simulink model "PI_v3"  (R2022b)
settings: Solver=FixedStepAuto  StartTime=0.0  StopTime=250  FixedStep=0.1  RelTol=1e-3  EnableMultiTasking=on
InitFcn:
  | Ts = 0.1
values from neighbouring files (symbols this model uses):
  ki = 10^controllerParams(2)    [objFunDreitankt.m]
  kp = 10^controllerParams(1)    [objFunDreitankt.m]
  tstart = min(simout.enableControl.time(simout.enableControl.signals.values > 0.5))    [objFunDreitankt.m]
  upperBound1stank = 7.5*10^-3    (= 0.0075)    [objFunDreitankt.m]
  V101_ref = 0    [objFunDreitankt.m]
undefined symbols (not defined in the file or in its folder): ESSettings, f, Parameters
libraries: etargetslib x134, simulink x32, instrumentlib x2, pid_lib x1, slpidlib x1, UtilLib x1
settings Model: Creator=ST  LastModifiedBy=vd818225
settings SolverCC: ZeroCrossAlgorithm=Adaptive  AlgebraicLoopSolver=TrustRegion  AutoInsertRateTranBlk=on
settings DataIOCC: LimitDataPoints=on  SaveFormat=Array  ReturnWorkspaceOutputs=off
settings OptimizationCC: LifeSpan=inf
settings DebuggingCC: UnderspecifiedInitializationDetection=Classic  MergeDetectMultiDrivingBlocksExec=none  SolverPrmCheckMsg=warning  UnconnectedInputMsg=warning  UnconnectedOutputMsg=warning  UnconnectedLineMsg=warning  StateNameClashWarn=warning  SFUnexpectedBacktrackingDiag=warning  SFNoUnconditionalDefaultTransitionDiag=warning  SFExecutionAtInitializationDiag=none  SFMachineParentedDataDiag=warning  ArithmeticOperatorsInVariantConditions=warning
settings HardwareCC: ProdBitPerPointer=32  ProdBitPerSizeT=32  ProdBitPerPtrDiffT=32  ProdLargestAtomicFloat=None  ProdIntDivRoundTo=Undefined  ProdEndianess=Unspecified  ProdWordSize=32  ProdHWDeviceType=32-bit Generic
settings ModelReferenceCC: EnableRefExpFcnMdlSchedulingChecks=on  PropagateSignalLabelsOutOfModel=off
settings SFSimCC: SimUseLocalCustomCode=off  CustomCodeUndefinedFunction=UseInterfaceOnly
settings RTWCC: RTWUseLocalCustomCode=off  DLArmComputeVersion=19.05
settings CodeAppCC: StateflowObjectComments=on
settings GRTTargetCC: TargetLangStandard=C89/C90 (ANSI)
settings ConfigComp: CovMetricSettings=dw  CovSaveCumulativeToWorkspaceVar=on  CovSaveSingleToWorkspaceVar=on  CovExternalEMLEnable=off  CovSFcnEnable=off

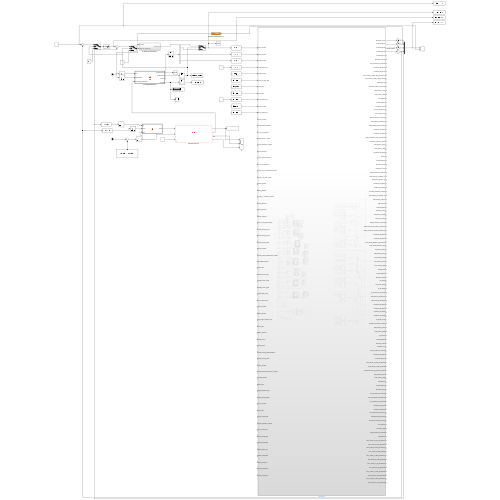
[thumbnail: Simulink's stored preview of the top-level diagram]
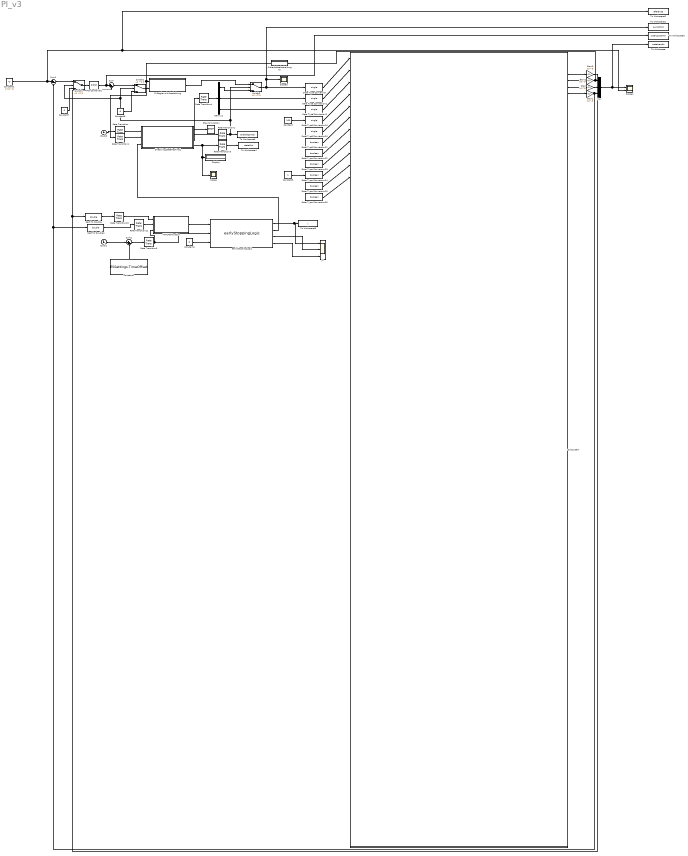
== system PI_v3 ==
  Cast To Double : DataTypeConversion  OutDataTypeStr=double  SaturateOnIntegerOverflow=off  RndMeth=Floor
  Cast To Double1 : DataTypeConversion  OutDataTypeStr=double  SaturateOnIntegerOverflow=off  RndMeth=Floor
  Clock1 : Clock
  Clock3 : Clock
  Constant : Constant  Value=100
  Constant1 : Constant  Value=4*10^-3
  Constant2 : Constant  Value=ESSettings.TimeOffset
  Constant3 : Constant
  Constant4 : Constant  Value=0
  Constant7 : Constant  Value=0
  Constant8 : Constant  Value=0
  Data Type Conversion{,1..2,19..20} (5 alike) : DataTypeConversion  OutDataTypeStr=single  SaturateOnIntegerOverflow=off  RndMeth=Floor
  Data Type Conversion{21..26} (6 alike) : DataTypeConversion  OutDataTypeStr=boolean  SaturateOnIntegerOverflow=off  RndMeth=Floor
  Demux1 : Demux  Outputs=3
  Display : Display
  Gain : Gain  Gain=10^-3
  Gain1 : Gain  Gain=10^-3
  Gain2 : Gain  Gain=10^-3
  Gain3 : Gain  Gain=10^-5
  J1 : Scope  NumInputPorts=3
  MATLAB Function : MATLAB Function  TreatAsAtomicUnit=on
  Mux : Mux  Inputs=3
  PI-Regler mit Abschaltung : Subsystem
  PID Controller1 : slpidlib/PID Controller  Controller=PID  Form=Parallel  TimeDomain=Continuous-time  UseExternalTs=off  SampleTime=-1  IntegratorMethod=Forward Euler  FilterMethod=Forward Euler  ControllerParametersSource=internal  P=kp  I=ki  UseKiTs=off  D=0  N=100  UseFilter=on  TunerSelectOption=Transfer Function Based (PID Tuner App)  InitialConditionSource=internal  InitialConditionForIntegrator=0  InitialConditionForFilter=0  DifferentiatorICPrevScaledInput=0  ExternalReset=none  TrackingMode=off  Kt=1  LimitOutput=on  SatLimitsSource=internal  UpperSaturationLimit=50/60  LowerSaturationLimit=0  LinearizeAsGain=on  AntiWindupMode=clamping  Kb=1  LimitIntegrator=off  UpperIntegratorSaturationLimit=inf  LowerIntegratorSaturationLimit=-inf  POutMin=[]  POutMax=[]  IOutMin=[]  IOutMax=[]  DOutMin=[]  DOutMax=[]  NOutMin=[]  NOutMax=[]  SumOutMin=[]  SumOutMax=[]  SaturationOutMin=[]  SaturationOutMax=[]  PParamMin=[]  PParamMax=[]  IParamMin=[]  IParamMax=[]  DParamMin=[]  DParamMax=[]  NParamMin=[]  NParamMax=[]  KbParamMin=[]  KbParamMax=[]  KtParamMin=[]  KtParamMax=[]  KbOutMin=[]  KbOutMax=[]  KtOutMin=[]  KtOutMax=[]  IntegratorOutMin=[]  IntegratorOutMax=[]  FilterOutMin=[]  FilterOutMax=[]  SumI1OutMin=[]  SumI1OutMax=[]  SumI2OutMin=[]  SumI2OutMax=[]  SumI3OutMin=[]  SumI3OutMax=[]  SumI4OutMin=[]  SumI4OutMax=[]  SumDOutMin=[]  SumDOutMax=[]  DifferentiatorOutMin=[]  DifferentiatorOutMax=[]  FilterDiffOutCoefMin=[]  FilterDiffOutCoefMax=[]  ReciprocalOutMin=[]  ReciprocalOutMax=[]  SumDenOutMin=[]  SumDenOutMax=[]  SumNumOutMin=[]  SumNumOutMax=[]  DivideOutMin=[]  DivideOutMax=[]  UdiffTsProdOutMin=[]  UdiffTsProdOutMax=[]  NTsProdOutMin=[]  NTsProdOutMax=[]  UintegralTsProdOutMin=[]  UintegralTsProdOutMax=[]  UngainTsProdOutMin=[]  UngainTsProdOutMax=[]  ClampingZeroOutDataTypeStr=Inherit: Inherit via back propagation  ClampingZeroOutMin=[]  ClampingZeroOutMax=[]  FilterDenConstantOutDataTypeStr=Inherit: Inherit via back propagation  FilterDenConstantOutMin=[]  FilterDenConstantOutMax=[]  PCopyOutDataTypeStr=Inherit: Inherit via back propagation  PCopyOutMin=[]  PCopyOutMax=[]  NCopyOutDataTypeStr=Inherit: Inherit via back propagation  NCopyOutMin=[]  NCopyOutMax=[]  IntegratorContinuousStateAttributes=''  IntegratorStateMustResolveToSignalObject=off  IntegratorRTWStateStorageClass=Auto  FilterContinuousStateAttributes=''  FilterStateMustResolveToSignalObject=off  FilterRTWStateStorageClass=Auto  ParallelPVariant=InternalParameters  IdealPVariant=Disabled  IVariant=InternalParameters  DVariant=InternalParameters  IntegratorVariant=Continuous  SatVariant=Enabled  AWVariant=ContClampingParallel  PCopyVariant=Disabled  TRVariant=Disabled  FdbkBlocksVariant=Forward  IdealPFdbkVariant=Disabled  SatFdbkVariant=Disabled  DerivativeFilterVariant=ContFilter  NVariant=InternalParameters  NCopyVariant=Disabled  FilterICVariant=InternalICsFilter  IntegratorICVariant=InternalICs  ExternalResetVariant=Disabled  TRSumVariant=Passthrough  SumFdbkVariant=Disabled  SumVariant=Sum_PID  TsampFilterVariant=InternalTs  TsampNgainVariant=Passthrough  TsampIntegralVariant=Passthrough  ExternalSaturationOutDataTypeStr=Inherit: Same as second input
  Rate Transition : RateTransition  OutPortSampleTime=0.1
  Rate Transition1 : RateTransition  OutPortSampleTime=0.1
  Rate Transition10 : RateTransition  OutPortSampleTime=ESSettings.t_obj
  Rate Transition11 : RateTransition  OutPortSampleTime=ESSettings.t_obj
  Rate Transition2 : RateTransition
  Rate Transition3 : RateTransition
  Rate Transition4 : RateTransition
  Rate Transition9 : RateTransition  OutPortSampleTime=ESSettings.t_obj
  Scope : Scope
  Scope1 : Scope  NumInputPorts=2
  Scope3 : Scope
  ShedulingStateMachine1 : MATLAB Function  TreatAsAtomicUnit=on
  Sicherheitsabschaltung V2 : Subsystem
  Stop Simulation : Stop
  Subsystem : Subsystem
  Sum : Sum  Inputs=|+-
  Sum1 : Sum  Inputs=|+-
  Sum2 : Sum  Inputs=|+-
  Switch1 : Switch  Criteria=u2 ~= 0  Threshold=tstart  SaturateOnIntegerOverflow=off  InputSameDT=off
  Switch2 : Switch  Criteria=u2 ~= 0  Threshold=tstart  SaturateOnIntegerOverflow=off  InputSameDT=off
  Switch3 : Switch  Criteria=u2 ~= 0  Threshold=tstart  SaturateOnIntegerOverflow=off  InputSameDT=off
  To Workspace : ToWorkspace  VariableName=waterLevels  SaveFormat=Structure With Time  SampleTime=-1
  To Workspace1 : ToWorkspace  VariableName=pumpCmd  SaveFormat=Structure With Time  SampleTime=-1
  To Workspace2 : ToWorkspace  VariableName=reference  SaveFormat=Structure With Time  SampleTime=-1
  To Workspace3 : ToWorkspace  VariableName=outerLoopCmd  SaveFormat=Structure With Time  SampleTime=-1
  To Workspace4 : ToWorkspace  VariableName=stateOut  SaveFormat=Structure With Time  SampleTime=-1
  To Workspace5 : ToWorkspace  VariableName=enableControl  SaveFormat=Structure With Time  SampleTime=-1
  To Workspace8 : ToWorkspace  VariableName=j  SaveFormat=Structure With Time  SampleTime=-1
  earlyStoppingLogic : UtilLib/earlyStoppingLogic  SystemSampleTime=-1  VariantActivationTime=update diagram  Latency=0  AutoFrameSizeCalculation=off
  wires:
  Data Type Conversion2/1 -> Subsystem/3(V106_Stellwert)
  Data Type Conversion/1 -> Subsystem/1(P101_Stellwert)
  Data Type Conversion1/1 -> Subsystem/2(V101_Stellwert)
  Data Type Conversion19/1 -> Subsystem/4(V106_Aktivierung)
  Data Type Conversion20/1 -> Subsystem/5(P102_Stellwert)
  Data Type Conversion21/1 -> Subsystem/6(V107_zu_KMP_VBS)
  Data Type Conversion22/1 -> Subsystem/7(V101_offen)
  Data Type Conversion23/1 -> Subsystem/8(V106_offen)
  Data Type Conversion24/1 -> Subsystem/9(P101_Aktivierung)
  Data Type Conversion25/1 -> Subsystem/10(V105_zu_VBS)
  Data Type Conversion26/1 -> Subsystem/11(P102_Aktivierung)
  Sicherheitsabschaltung V2/1(Notaus) -> Rate Transition1/1, PI-Regler mit Abschaltung/1(Not-Aus)
  PID Controller1/1 -> To Workspace3/1, Sum/1
  Sum1/1 -> Switch1/1
  Constant/1 -> Data Type Conversion19/1
  Constant3/1 -> Data Type Conversion24/1
  Subsystem/4(Fuellstand_B104) -> Gain1/1
  Subsystem/3(Fuellstand_B103) -> Gain/1  "Fuellstand_B103"
  Subsystem/2(Fuellstand_B102) -> Gain2/1
  Subsystem/1(Durchfluss_FI101) -> Gain3/1
  Gain2/1 -> Sicherheitsabschaltung V2/1(V2), Mux/1
  Gain/1 -> Mux/2
  Mux/1 -> To Workspace/1, Scope1/1
  Demux1/2 -> Data Type Conversion1/1
  Switch3/1 -> Data Type Conversion/1, To Workspace1/1, Scope3/1
  Demux1/3 -> Data Type Conversion2/1
  Constant1/1 -> To Workspace2/1, Scope1/2, Sum1/1
  Constant7/1 -> Switch1/3
  Switch1/1 -> PID Controller1/1
  Switch2/1 -> PI-Regler mit Abschaltung/2(Q_P101_soll [m^3/s])
  Rate Transition2/1 -> To Workspace5/1, Switch1/2, Switch2/2, Switch3/2
  Constant8/1 -> Switch2/3
  ShedulingStateMachine1/2(enableControl) -> Rate Transition2/1
  Sum/1 -> Switch2/1
  Clock3/1 -> Rate Transition/1
  ShedulingStateMachine1/1(stopExperiment) -> Stop Simulation/1
  Demux1/1 -> Switch3/3
  ShedulingStateMachine1/4(stateOut) -> Rate Transition3/1, Scope/1, Display/1
  PI-Regler mit Abschaltung/1(U_P101 [%]) -> Switch3/1
  Rate Transition/1 -> ShedulingStateMachine1/1(time)
  Rate Transition1/1 -> ShedulingStateMachine1/2(notAusActive)
  Rate Transition3/1 -> To Workspace4/1
  ShedulingStateMachine1/3(sollVals) -> Rate Transition4/1
  Rate Transition4/1 -> Demux1/1
  Sum2/1 -> Rate Transition9/1
  Gain3/1 -> Cast To Double/1, Sum/2
  Constant4/1 -> earlyStoppingLogic/3
  Rate Transition9/1 -> MATLAB Function/3(time), earlyStoppingLogic/2
  earlyStoppingLogic/2 -> ShedulingStateMachine1/3(earlyStoppingActivated)
  earlyStoppingLogic/3 -> J1/2  "JOut"
  Rate Transition11/1 -> MATLAB Function/2(meas)
  Rate Transition10/1 -> MATLAB Function/1(ref)
  MATLAB Function/1(ITAE) -> earlyStoppingLogic/1
  Clock1/1 -> Sum2/1
  Constant2/1 -> Sum2/2
  earlyStoppingLogic/4 -> J1/3
  Gain1/1 -> Cast To Double1/1, Sum1/2, Mux/3
  earlyStoppingLogic/1 -> J1/1, To Workspace8/1
  Cast To Double/1 -> Rate Transition10/1
  Cast To Double1/1 -> Rate Transition11/1

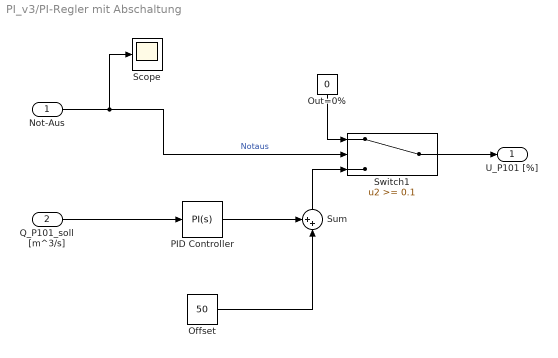
== system PI_v3/PI-Regler mit Abschaltung ==
  Not-Aus : Inport
  Q_P101_soll [m^3/s] : Inport  Port=2
  Offset : Constant  Value=50
  Out=0% : Constant  Value=0
  PID Controller : pid_lib/PID Controller  Controller=PI  Form=Parallel  TimeDomain=Continuous-time  UseExternalTs=off  SampleTime=-1  IntegratorMethod=Forward Euler  FilterMethod=Forward Euler  ControllerParametersSource=internal  P=30e3  I=0.6e3  D=0  UseFilter=on  N=100  TunerSelectOption=Transfer Function Based (PID Tuner App)  InitialConditionSource=internal  InitialConditionForIntegrator=0  InitialConditionForFilter=0  DifferentiatorICPrevScaledInput=0  ExternalReset=none  TrackingMode=off  Kt=1  LimitOutput=on  SatLimitsSource=internal  UpperSaturationLimit=50  LowerSaturationLimit=-50  LinearizeAsGain=on  AntiWindupMode=clamping  Kb=1  POutMin=[]  POutMax=[]  IOutMin=[]  IOutMax=[]  DOutMin=[]  DOutMax=[]  NOutMin=[]  NOutMax=[]  SumOutMin=[]  SumOutMax=[]  SaturationOutMin=[]  SaturationOutMax=[]  PParamMin=[]  PParamMax=[]  IParamMin=[]  IParamMax=[]  DParamMin=[]  DParamMax=[]  NParamMin=[]  NParamMax=[]  KbParamMin=[]  KbParamMax=[]  KtParamMin=[]  KtParamMax=[]  KbOutMin=[]  KbOutMax=[]  KtOutMin=[]  KtOutMax=[]  IntegratorOutMin=[]  IntegratorOutMax=[]  FilterOutMin=[]  FilterOutMax=[]  SumI1OutMin=[]  SumI1OutMax=[]  SumI2OutMin=[]  SumI2OutMax=[]  SumI3OutMin=[]  SumI3OutMax=[]  SumI4OutMin=[]  SumI4OutMax=[]  SumDOutMin=[]  SumDOutMax=[]  DifferentiatorOutMin=[]  DifferentiatorOutMax=[]  FilterDiffOutCoefMin=[]  FilterDiffOutCoefMax=[]  ReciprocalOutMin=[]  ReciprocalOutMax=[]  SumDenOutMin=[]  SumDenOutMax=[]  SumNumOutMin=[]  SumNumOutMax=[]  DivideOutMin=[]  DivideOutMax=[]  UdiffTsProdOutMin=[]  UdiffTsProdOutMax=[]  NTsProdOutMin=[]  NTsProdOutMax=[]  UintegralTsProdOutMin=[]  UintegralTsProdOutMax=[]  UngainTsProdOutMin=[]  UngainTsProdOutMax=[]  IntegratorContinuousStateAttributes=''  IntegratorStateMustResolveToSignalObject=off  IntegratorRTWStateStorageClass=Auto  FilterContinuousStateAttributes=''  FilterStateMustResolveToSignalObject=off  FilterRTWStateStorageClass=Auto  ParallelPVariant=InternalParameters  IdealPVariant=Disabled  IVariant=InternalParameters  DVariant=Disabled  IntegratorVariant=Continuous  SatVariant=Enabled  AWVariant=ContClampingParallel  PCopyVariant=Disabled  TRVariant=Disabled  FdbkBlocksVariant=Forward  IdealPFdbkVariant=Disabled  SatFdbkVariant=Disabled  DerivativeFilterVariant=Disabled  NVariant=Disabled  NCopyVariant=Disabled_SignalSpec  FilterICVariant=Disabled  IntegratorICVariant=InternalICs  ExternalResetVariant=Disabled  TRSumVariant=Passthrough  SumFdbkVariant=Disabled  SumVariant=Sum_PI  TsampFilterVariant=InternalTs  TsampNgainVariant=Passthrough  TsampIntegralVariant=Passthrough  ExternalSaturationOutDataTypeStr=Inherit: Same as second input
  Scope : Scope
  Sum : Sum  Inputs=++|
  Switch1 : Switch  Threshold=0.1
  U_P101 [%] : Outport
  wires:
  Q_P101_soll [m^3/s]/1 -> PID Controller/1
  Switch1/1 -> U_P101 [%]/1
  Out=0%/1 -> Switch1/1
  Not-Aus/1 -> Scope/1, Switch1/2  "Notaus"
  Sum/1 -> Switch1/3
  PID Controller/1 -> Sum/1
  Offset/1 -> Sum/2

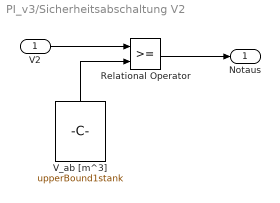
== system PI_v3/Sicherheitsabschaltung V2 ==
  V2 : Inport
  Relational Operator : RelationalOperator  InputSameDT=off
  V_ab [m^3] : Constant  Value=upperBound1stank
  Notaus : Outport
  wires:
  V2/1 -> Relational Operator/1
  V_ab [m^3]/1 -> Relational Operator/2
  Relational Operator/1 -> Notaus/1

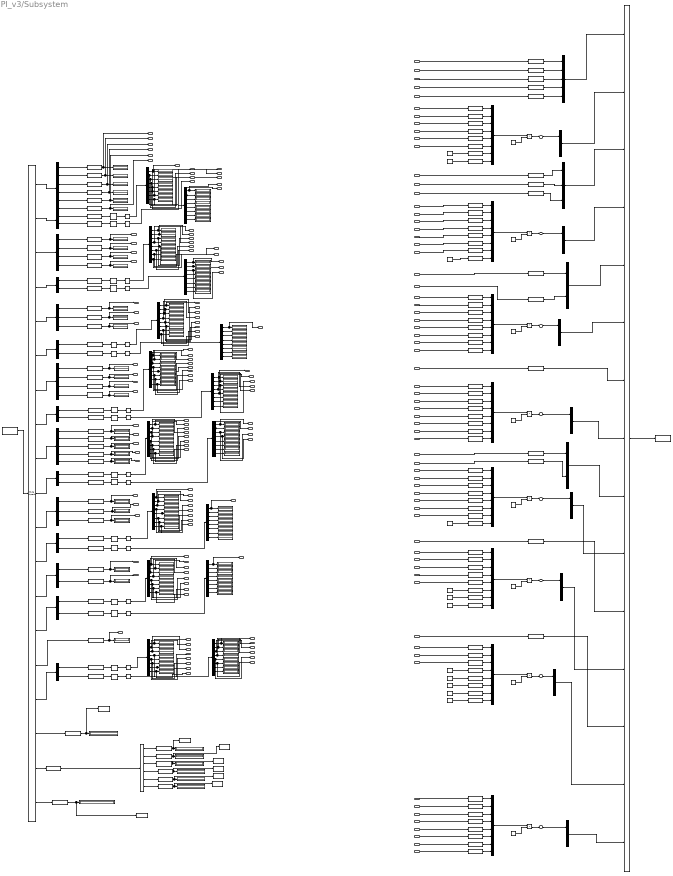
== system PI_v3/Subsystem ==
  P101_Stellwert : Inport
  V101_Stellwert : Inport  Port=2
  V106_Stellwert : Inport  Port=3
  V106_Aktivierung : Inport  Port=4
  P102_Stellwert : Inport  Port=5
  V107_zu_KMP_VBS : Inport  Port=6
  V101_offen : Inport  Port=7
  V106_offen : Inport  Port=8
  P101_Aktivierung : Inport  Port=9
  V105_zu_VBS : Inport  Port=10
  P102_Aktivierung : Inport  Port=11
  P201_Stellwert : Inport  Port=12
  V206_Wasser_Stellwert : Inport  Port=13
  V211_Gas_Stellwert : Inport  Port=14
  V202_Ablauf_zu_REH : Inport  Port=15
  V207_Ruecklauf_zu_B201 : Inport  Port=16
  P201_aktivieren : Inport  Port=17
  V206_Wasser_aktivieren : Inport  Port=18
  V211_Gas_aktivieren : Inport  Port=19
  V204_nach_Druckbehaelter_drehen : Inport  Port=20
  V205_nach_VBS_drehen : Inport  Port=21
  P301_Stellwert : Inport  Port=22
  R304_Stellwert : Inport  Port=23
  V305_zu_umwaelzen_oeffnen : Inport  Port=24
  W303_aktivieren : Inport  Port=25
  P301_aktivieren : Inport  Port=26
  R304_aktivieren : Inport  Port=27
  V307_Zulauf_REK_oeffnen : Inport  Port=28
  V306_Stellung_extern : Inport  Port=29
  V304_Stellung_extern : Inport  Port=30
  V305_Stellung_VBS : Inport  Port=31
  P401_Stellwert : Inport  Port=32
  V402_Ablauf_Kuehlbehaelter_oeffnen : Inport  Port=33
  Kuehlkreislauf_aktiv : Inport  Port=34
  P401_aktiv : Inport  Port=35
  V406_kuehlen_klein : Inport  Port=36
  V406_kuehlen_mittel : Inport  Port=37
  V406_kuehlen_gross : Inport  Port=38
  V405_VBS_drehen : Inport  Port=39
  V411_VBS_drehen : Inport  Port=40
  P501_Stellwert : Inport  Port=41
  R504_Stellwert : Inport  Port=42
  pH_Regler_schalten_hold : Inport  Port=43
  P501_aktiv : Inport  Port=44
  R504_aktivieren : Inport  Port=45
  V502_Saeure : Inport  Port=46
  V503_Lauge : Inport  Port=47
  V504_Stellung_Nachfolgestation : Inport  Port=48
  V505_Stellung_VBS1 : Inport  Port=49
  P601_Stellwert : Inport  Port=50
  V602_Ablauf_Kuehlbehaeler_oeffnen : Inport  Port=51
  V604_Ruecklauf : Inport  Port=52
  P601_aktiv : Inport  Port=53
  P602_Abfuellen_aktiv : Inport  Port=54
  V605_Stellung_VBS1 : Inport  Port=55
  P701_Stellwert : Inport  Port=56
  P701_aktiv : Inport  Port=57
  V701_Zulauf_B701 : Inport  Port=58
  V702_Ruecklauf_zu_B701 : Inport  Port=59
  V911_Zulauf_MTL : Inport  Port=60
  V921_Zulauf_KMP : Inport  Port=61
  V941_Zulauf_REK : Inport  Port=62
  P901_Aktivierung : Inport  Port=63
  V931_Zulauf_REH : Inport  Port=64
  V951_Zulauf_PH : Inport  Port=65
  V961_Zulauf_ZWL : Inport  Port=66
  V971_Zulauf_RCY : Inport  Port=67
  AI_pH_QI502_PB_DATABASE : Display
  B101_Fuellstand : Display
  B102_Fuellstand : Display
  B103_Fuellstand : Display
  B104_Fuellstand : Display
  B201_Fuellstand : Display
  B501_Fuellstand : Display
  B601_Fuellstand_LI610 : Display
  B701_Fuellstand_B701_LI701 : Display
  Bitwise AND{,1..15} (16 alike) : simulink/Logic and Bit Operations/Bitwise Operator  logicop=AND  UseBitMask=on  BitMask=uint8([1;2;4;8;16;32;64;128])  BitMaskRealWorld=Stored Integer
  Byte Pack1 : etargetslib/Byte Pack  datatypes={'single','uint8','single','uint8','single','uint8','single','uint8','single','uint8','single','uint8','single','uint8','uint8'}  byteAlign=1
  Byte Reversal{80..211} (132 alike) : etargetslib/Byte Reversal  numInp=1
  Byte Unpack : etargetslib/Byte Unpack  dimensions={6,2,4,2,3,2,4,2,5,2,3,2,2,2,1,2,1,6,1}  datatypes={'single','uint8','single','uint8','single','uint8','single','uint8','single','uint8','single','uint8','single','uint8','single','uint8','uint16','uint8','uint32'}  byteAlign=1
  Byte Vektor{8..15} (8 alike) : Constant  Value=[1,2,4,8,16,32,64,128]  OutDataTypeStr=single
  Compare To Constant{,1..15} (16 alike) : simulink/Logic and Bit Operations/Compare To Constant  relop=~=  const=0  OutDataTypeStr=uint8
  Data Type Conversion{,1..7} (8 alike) : DataTypeConversion  OutDataTypeStr=single  SaturateOnIntegerOverflow=off  RndMeth=Floor
  Demux : Demux  Outputs=6
  Demux{1..3,8..9,12..13,16..17,20..21,24..25,28..30} (16 alike) : Demux  Outputs=8
  Demux10 : Demux  Outputs=3
  Demux{5,7,11,15,19,23,26..27,31} (9 alike) : Demux  Outputs=2
  Demux14 : Demux
  Demux18 : Demux  Outputs=5
  Demux22 : Demux  Outputs=3
  Demux4 : Demux  Outputs=6
  Demux6 : Demux
  Durchfluss FI301 : Display
  Durchfluss FI401 : Display
  Durchfluss_VBS_1 : Display
  FI101_Durchfluss : Display
  FI501_Durchflussmessung : Display
  FI601_Durchflussmessung : Display
  FI701_Durchflussmessung : Display
  FIC102_Durchfluss_B202 : Display
  FL201_Durchfluss : Display
  Fuellbit : Constant  Value=0  OutDataTypeStr=boolean
  Fuellbit1 : Constant  Value=0  OutDataTypeStr=boolean
  Füllstand B{1..128,301,401} (130 alike) : Display
  Mux{1..2,24..25,27..28,30,32} (8 alike) : Mux  Inputs=8
  Mux{3,12,14..19,26,33} (10 alike) : Mux  Inputs=2
  Mux29 : Mux  Inputs=5
  Mux31 : Mux  Inputs=3
  Nicht belegt {14..16,18..24} (10 alike) : Constant  Value=0  OutDataTypeStr=boolean
  PI201_Druck_Gas : Display
  PI202_Druck_Wasser : Display
  Product{8..15} (8 alike) : Product
  QI502_pH_Messung_in_B504 : Display
  T501_Temperatur{3..8} (6 alike) : Display
  TI503_Temperaturmessung_in_B504 : Display
  Temperature T301 : Display
  Temperature TI401 : Display
  Temperature TIx Temperaturumschalter : Display
  UDP Receive1 : instrumentlib/UDP Receive  Priority=3  Host=134.130.45.33  Port=2000  LocalPort=2000  EnablePortSharing=off  GetLatestData=on  DataSize=140  DataType=uint8  ASCIIFormatting=%f,  Terminator=LF  ByteOrder=BigEndian  EnableBlockingMode=on  Timeout=5  SampleTime=0.1  LocalAddress=134.130.45.62
  UDP Send2 : instrumentlib/UDP Send  Priority=2  Host=134.130.45.33  Port=2001  LocalPort=2001  EnablePortSharing=off  ByteOrder=BigEndian  OutputDatagramPacketSize=74  EnableBlockingMode=on  LocalAddress=134.130.45.62
  Vektor Summe{8..15} (8 alike) : Sum  Inputs=1  OutDataTypeStr=uint8
  WI620_Gewichtsmessung : Display
  nanosecond : Display
  year : Display
  Durchfluss_FI101 : Outport
  Fuellstand_B102 : Outport  Port=2
  Fuellstand_B103 : Outport  Port=3
  Fuellstand_B104 : Outport  Port=4
  Fuellstand_B101 : Outport  Port=5
  Durchfluss_FIC102 : Outport  Port=6
  MTL_Drucksensor_Druckluft : Outport  Port=7
  Fuellstand_Max_B101 : Outport  Port=8
  Fuellstand_Min_B101 : Outport  Port=9
  V102_Ablauf_zu_KMP_VBS_geschlossen : Outport  Port=10
  V102_Ablauf_zu_KMP_VBS_geoeffnet : Outport  Port=11
  Stoerung_P101 : Outport  Port=12
  Durchfluss_FIC101_Grenzwert : Outport  Port=13
  V105_Stellung_intern : Outport  Port=14
  V105_Stellung_VBS : Outport  Port=15
  MTL_Notaus : Outport  Port=16
  Fuellstand_B201 : Outport  Port=17
  Durchfluss_FL201 : Outport  Port=18
  Druck_Pi202_Wasser : Outport  Port=19
  Druck_Pi201_Gas : Outport  Port=20
  KMP_Drucksensor_Druckluft : Outport  Port=21
  V204_Stellung_Umwaelzen : Outport  Port=22
  V204_Stellung_Druckbehaelter : Outport  Port=23
  Fuellstand_Max_B201 : Outport  Port=24
  Fuellstand_Min_B201 : Outport  Port=25
  KMP_Drucksensor_Gas_Schwellwert : Outport  Port=26
  Druchfluss_Grenzwert_FI201 : Outport  Port=27
  V205_Stellung_intern : Outport  Port=28
  V205_Stellung_VBS : Outport  Port=29
  Fuellstand_Max_B202 : Outport  Port=30
  Notaus : Outport  Port=31
  Fuellstand_B301 : Outport  Port=32
  Durchfluss_FI301 : Outport  Port=33
  Temperatur_T301 : Outport  Port=34
  REH_Drucksensor_Druckluft : Outport  Port=35
  V304_Stellung_umwaelzen_in : Outport  Port=36
  V304_Stellung_extern_in : Outport  Port=37
  Fuellstand_Max_B301 : Outport  Port=38
  Fuellstand_Min_B301 : Outport  Port=39
  Durchfluss_Grenzwert_FIC301 : Outport  Port=40
  V305_Stellung_Folgestation_in : Outport  Port=41
  V305_Stellung_VBS_in : Outport  Port=42
  REH_Notaus : Outport  Port=43
  Fuellstand_B401 : Outport  Port=44
  Durchfluss_FI401 : Outport  Port=45
  Temperatur_TIx_REK : Outport  Port=46
  Temperatur_TI401 : Outport  Port=47
  REK_Drucksensor_Druckluft : Outport  Port=48
  Nieder_Hochdruck_Schalter_Hochdruck : Outport  Port=49
  Nieder_Hochdruck_Schalter_Niederdruck : Outport  Port=50
  Fuellstand_Max_B401 : Outport  Port=51
  Fuellstand_Min_B401 : Outport  Port=52
  V402_Ablauf_Behaelter_geschlossen : Outport  Port=53
  V402_Ablauf_Behaelter_offen : Outport  Port=54
  Durchfluss_FIC401 : Outport  Port=55
  V405_Stellung_intern : Outport  Port=56
  V405_Stellung_REH : Outport  Port=57
  V411_Stellung_intern : Outport  Port=58
  V411_Stellung_VBS : Outport  Port=59
  REK_Notaus : Outport  Port=60
  Fuellstand_B501 : Outport  Port=61
  Durchfluss_FI501 : Outport  Port=62
  pH_QI502 : Outport  Port=63
  Temperatur_TI503 : Outport  Port=64
  pH_AI_QI502 : Outport  Port=65
  pH_Drucksensor_Druckluft : Outport  Port=66
  V504_Stellung_Umwaelzen : Outport  Port=67
  V504_Stellung_Nachfolger : Outport  Port=68
  Fuellstand_Max_B501 : Outport  Port=69
  Fuellstand_Min_B501 : Outport  Port=70
  Fuellstand_Min_B502 : Outport  Port=71
  Fuellstand_Min_B503 : Outport  Port=72
  pH_Regler_A517 : Outport  Port=73
  Durchfluss_Grenzwert_FIC501 : Outport  Port=74
  V505_Stellung_intern : Outport  Port=75
  V505_Stellung_VBS : Outport  Port=76
  pH_Notaus : Outport  Port=77
  Fuellstand_B601 : Outport  Port=78
  Durchfluss_FI601 : Outport  Port=79
  Durchfluss_FI1 : Outport  Port=80
  ZWL_Drucksensor_druckluft : Outport  Port=81
  Fuellstand_Max_B601 : Outport  Port=82
  Fuellstand_Min_B1 : Outport  Port=83
  V602_Ablauf_zu_ABF_geschlossen : Outport  Port=84
  V602_Ablauf_zu_ABF_geoeffnet : Outport  Port=85
  Durchflussmessung_Grenzwert_FIC601 : Outport  Port=86
  V605_Stellung_intern : Outport  Port=87
  V605_Stellung_VBS : Outport  Port=88
  ZWL_Notaus : Outport  Port=89
  Fuellstand_B701 : Outport  Port=90
  Durchfluss_FI701 : Outport  Port=91
  RCY_Drucksensor_Druckluft : Outport  Port=92
  V701_Zulauf_B701_geschlossen : Outport  Port=93
  V701_Zulauf_B701_geoeffnet : Outport  Port=94
  Fuellstand_Max_B701 : Outport  Port=95
  Fuellstand_Min_B701 : Outport  Port=96
  V702_Ruecklauf_geschlossen : Outport  Port=97
  V702_Ruecklauf_geoeffnet : Outport  Port=98
  Durchfluss_Grenzwert_FIC701 : Outport  Port=99
  RCY_Notaus : Outport  Port=100
  Durchfluss_VBS : Outport  Port=101
  VBS_Drucksensor_Druckluft : Outport  Port=102
  VBS_Notaus : Outport  Port=103
  V911_Zulauf_zu_MTL_geschlossen : Outport  Port=104
  V911_Zulauf_zu_MTL_geoeffnet : Outport  Port=105
  V911_Zulauf_zu_KMP_geschlossen : Outport  Port=106
  V911_Zulauf_zu_KMP_geöffnet : Outport  Port=107
  V911_Zulauf_zu_REH_geschlossen : Outport  Port=108
  V911_Zulauf_zu_REH_geoeffnet : Outport  Port=109
  V911_Zulauf_zu_pH_geschlossen : Outport  Port=110
  V911_Zulauf_zu_pH_geoeffnet : Outport  Port=111
  V911_Zulauf_zu_ZWL_geschlossen : Outport  Port=112
  V911_Zulauf_zu_ZWL_geoeffnet : Outport  Port=113
  V911_Zulauf_zu_RCY_geschlossen : Outport  Port=114
  V911_Zulauf_zu_RCY_geoeffnet : Outport  Port=115
  wires:
  Demux20/3 -> Fuellstand_Min_B1/1, Füllstand B83/1
  Demux12/7 -> V402_Ablauf_Behaelter_offen/1, Füllstand B55/1
  Demux12/6 -> V402_Ablauf_Behaelter_geschlossen/1, Füllstand B54/1
  Demux21/7 -> Füllstand B93/1
  Demux30/6 -> Füllstand B38/1
  Demux13/1 -> V405_Stellung_intern/1, Füllstand B63/1
  Demux9/4 -> Füllstand B26/1
  Demux15/2 -> Byte Reversal100/1
  Demux30/3 -> Füllstand B35/1
  Demux9/8 -> Füllstand B30/1
  Demux30/8 -> Füllstand B40/1
  Byte Reversal85/1 -> Fuellstand_B102/1, B102_Fuellstand/1
  Demux17/6 -> Füllstand B76/1
  Demux16/6 -> Fuellstand_Min_B502/1, Füllstand B70/1
  Compare To Constant10/1 -> Demux20/1
  Demux29/6 -> V911_Zulauf_zu_RCY_geoeffnet/1, Füllstand B124/1
  Demux16/8 -> pH_Regler_A517/1, Füllstand B72/1
  Compare To Constant4/1 -> Demux9/1
  Byte Unpack/12 -> Demux23/1
  Demux27/2 -> Byte Reversal117/1
  Demux3/8 -> Füllstand B7/1
  Byte Reversal86/1 -> Durchfluss_FL201/1, FL201_Durchfluss/1
  Demux13/6 -> Füllstand B60/1
  Demux24/5 -> Fuellstand_Min_B701/1, Füllstand B101/1
  Byte Reversal92/1 -> Temperatur_T301/1, Temperature T301/1
  Demux10/2 -> Byte Reversal91/1
  Byte Unpack/7 -> Demux14/1
  Byte Reversal121/1 -> Bitwise AND14/1
  Demux6/3 -> Byte Reversal87/1
  Compare To Constant/1 -> Demux1/1
  Demux7/2 -> Byte Reversal88/1
  Demux8/1 -> KMP_Drucksensor_Druckluft/1, Füllstand B32/1
  Demux20/4 -> V602_Ablauf_zu_ABF_geschlossen/1, Füllstand B84/1
  Demux25/8 -> Füllstand B110/1
  Demux16/4 -> Fuellstand_Max_B501/1, Füllstand B68/1
  Demux22/2 -> Byte Reversal110/1
  Byte Reversal88/1 -> Bitwise AND4/1
  Byte Reversal104/1 -> Durchfluss_FI501/1, FI501_Durchflussmessung/1
  Demux11/1 -> Byte Reversal93/1
  Demux20/8 -> V605_Stellung_VBS/1, Füllstand B88/1
  Byte Reversal123/1 -> Bitwise AND1/1
  Compare To Constant5/1 -> Demux30/1
  Demux30/1 -> REH_Notaus/1, Füllstand B48/1
  Byte Reversal81/1 -> Fuellstand_B201/1, B201_Fuellstand/1
  Demux21/4 -> Füllstand B90/1
  Demux17/2 -> V505_Stellung_intern/1, Füllstand B65/1
  Byte Reversal112/1 -> Bitwise AND11/1
  Demux2/6 -> Füllstand B14/1, Stoerung_P101/1
  Demux18/1 -> Byte Reversal102/1
  Demux9/3 -> Notaus/1, Füllstand B25/1
  Demux21/2 -> Füllstand B81/1
  Demux2/1 -> MTL_Drucksensor_Druckluft/1, Füllstand B9/1
  Byte Reversal122/1 -> Bitwise AND2/1
  Demux8/5 -> Fuellstand_Min_B201/1, Füllstand B21/1
  Demux20/5 -> V602_Ablauf_zu_ABF_geoeffnet/1, Füllstand B85/1
  Demux3/5 -> Füllstand B4/1
  Demux4/4 -> Byte Reversal83/1
  Demux12/1 -> REK_Drucksensor_Druckluft/1, Füllstand B64/1
  Demux3/1 -> V105_Stellung_VBS/1, Füllstand B8/1
  Demux17/8 -> Füllstand B78/1
  Demux24/6 -> V702_Ruecklauf_geschlossen/1, Füllstand B102/1
  Byte Reversal109/1 -> Fuellstand_B601/1, B601_Fuellstand_LI610/1
  Demux3/3 -> Füllstand B2/1
  Demux21/1 -> ZWL_Notaus/1, Füllstand B95/1
  Demux29/8 -> Füllstand B126/1
  Demux17/3 -> V505_Stellung_VBS/1, Füllstand B73/1
  Demux30/5 -> Füllstand B37/1
  Compare To Constant9/1 -> Demux17/1
  Demux8/2 -> V204_Stellung_Umwaelzen/1, Füllstand B18/1
  Demux24/4 -> Fuellstand_Max_B701/1, Füllstand B100/1
  Demux17/5 -> Füllstand B75/1
  Byte Reversal119/1 -> Durchfluss_VBS/1, Durchfluss_VBS_1/1
  Demux2/8 -> V105_Stellung_intern/1, Füllstand B16/1
  Byte Unpack/3 -> Demux6/1
  Demux5/2 -> Byte Reversal122/1
  Bitwise AND2/1 -> Compare To Constant2/1
  Byte Reversal115/1 -> Durchfluss_FIC102/1, FIC102_Durchfluss_B202/1
  Demux23/2 -> Byte Reversal112/1
  Demux4/3 -> Byte Reversal94/1
  Byte Reversal82/1 -> Druck_Pi201_Gas/1, PI201_Druck_Gas/1
  Byte Reversal91/1 -> Durchfluss_FI301/1, Durchfluss FI301/1
  Demux28/4 -> V911_Zulauf_zu_MTL_geoeffnet/1, Füllstand B116/1
  Bitwise AND3/1 -> Compare To Constant3/1
  Demux29/5 -> V911_Zulauf_zu_RCY_geschlossen/1, Füllstand B123/1
  Byte Reversal103/1 -> Temperatur_TI503/1, TI503_Temperaturmessung_in_B504/1
  Byte Unpack/16 -> Demux31/1
  Byte Reversal89/1 -> Bitwise AND3/1
  Demux26/2 -> Byte Reversal116/1
  Byte Reversal96/1 -> Fuellstand_B401/1, Füllstand B401/1
  Demux14/4 -> Byte Reversal97/1
  Demux12/8 -> Durchfluss_FIC401/1, Füllstand B56/1
  Compare To Constant6/1 -> Demux12/1
  Demux28/1 -> VBS_Drucksensor_Druckluft/1, Füllstand B128/1
  Byte Reversal98/1 -> Durchfluss_FI401/1, Durchfluss FI401/1
  Demux1/8 -> V305_Stellung_VBS_in/1, Füllstand B47/1
  Byte Unpack/1 -> Demux4/1
  Byte Reversal80/1 -> Durchfluss_FI101/1, FI101_Durchfluss/1
  Demux25/1 -> RCY_Notaus/1, Füllstand B111/1
  Demux17/4 -> pH_Notaus/1, Füllstand B74/1
  Byte Reversal118/1 -> Bitwise AND12/1
  Demux1/6 -> Durchfluss_Grenzwert_FIC301/1, Füllstand B45/1
  Demux30/2 -> Füllstand B34/1
  Demux13/5 -> REK_Notaus/1, Füllstand B59/1
  Bitwise AND13/1 -> Compare To Constant13/1
  Byte Reversal87/1 -> Druck_Pi202_Wasser/1, PI202_Druck_Wasser/1
  Demux26/1 -> Byte Reversal114/1
  Demux8/3 -> V204_Stellung_Druckbehaelter/1, Füllstand B19/1
  Compare To Constant7/1 -> Demux13/1
  Demux2/2 -> Fuellstand_Max_B101/1, Füllstand B10/1
  Demux13/2 -> V405_Stellung_REH/1, Füllstand B49/1
  Demux12/5 -> Fuellstand_Min_B401/1, Füllstand B53/1
  Demux11/2 -> Byte Reversal95/1
  Demux8/7 -> Druchfluss_Grenzwert_FI201/1, Füllstand B23/1
  Compare To Constant11/1 -> Demux21/1
  Demux9/2 -> Fuellstand_Max_B202/1, Füllstand B17/1
  Demux16/2 -> V504_Stellung_Umwaelzen/1, Füllstand B66/1
  Demux27/1 -> Byte Reversal118/1
  Demux4/2 -> Byte Reversal85/1
  Compare To Constant13/1 -> Demux25/1
  Demux22/3 -> Byte Reversal111/1
  Bitwise AND8/1 -> Compare To Constant8/1
  Compare To Constant14/1 -> Demux28/1
  Demux13/3 -> V411_Stellung_intern/1, Füllstand B57/1
  Demux25/6 -> Füllstand B108/1
  Byte Unpack/6 -> Demux11/1
  Demux24/8 -> Durchfluss_Grenzwert_FIC701/1, Füllstand B104/1
  Byte Reversal94/1 -> Fuellstand_B103/1, B103_Fuellstand/1
  Demux1/2 -> V304_Stellung_umwaelzen_in/1, Füllstand B41/1
  Bitwise AND5/1 -> Compare To Constant5/1
  Byte Reversal117/1 -> Bitwise AND13/1
  Demux3/7 -> Füllstand B6/1
  Bitwise AND/1 -> Compare To Constant/1
  Demux14/2 -> Byte Reversal98/1
  Compare To Constant3/1 -> Demux8/1
  Demux28/8 -> V911_Zulauf_zu_REH_geoeffnet/1, Füllstand B120/1
  Demux9/5 -> Füllstand B27/1
  Byte Unpack/2 -> Demux5/1
  Demux2/5 -> V102_Ablauf_zu_KMP_VBS_geoeffnet/1, Füllstand B13/1
  Byte Reversal83/1 -> B104_Fuellstand/1, Fuellstand_B104/1
  Demux31/2 -> Byte Reversal120/1
  Byte Reversal99/1 -> Temperatur_TIx_REK/1, Temperature TIx Temperaturumschalter/1
  Demux4/5 -> Byte Reversal84/1
  Demux14/3 -> Byte Reversal99/1
  Demux25/7 -> Füllstand B109/1
  Byte Reversal108/1 -> Bitwise AND8/1
  Demux10/1 -> Byte Reversal90/1
  Byte Unpack/10 -> Demux19/1
  Demux1/3 -> V304_Stellung_extern_in/1, Füllstand B42/1
  Bitwise AND12/1 -> Compare To Constant12/1
  Demux24/2 -> V701_Zulauf_B701_geschlossen/1, Füllstand B98/1
  Bitwise AND4/1 -> Compare To Constant4/1
  Byte Reversal90/1 -> Fuellstand_B301/1, Füllstand B301/1
  Demux3/4 -> Füllstand B3/1
  Demux1/4 -> Fuellstand_Max_B301/1, Füllstand B43/1
  Byte Reversal93/1 -> Bitwise AND/1
  Demux4/6 -> Byte Reversal115/1
  Demux10/3 -> Byte Reversal92/1
  Demux12/2 -> Nieder_Hochdruck_Schalter_Hochdruck/1, Füllstand B50/1
  Byte Reversal120/1 -> Bitwise AND15/1
  Demux21/8 -> Füllstand B94/1
  Demux8/4 -> Fuellstand_Max_B201/1, Füllstand B20/1
  Demux3/6 -> Füllstand B5/1
  Bitwise AND11/1 -> Compare To Constant11/1
  Byte Reversal95/1 -> Bitwise AND5/1
  Compare To Constant15/1 -> Demux29/1
  Byte Reversal113/1 -> Bitwise AND10/1
  Bitwise AND10/1 -> Compare To Constant10/1
  Demux29/2 -> V911_Zulauf_zu_pH_geoeffnet/1, Füllstand B113/1
  Byte Unpack/15 -> Byte Reversal119/1
  Demux1/1 -> REH_Drucksensor_Druckluft/1, Füllstand B33/1
  Demux9/7 -> Füllstand B29/1
  Demux12/4 -> Fuellstand_Max_B401/1, Füllstand B52/1
  Demux21/5 -> Füllstand B91/1
  Demux25/4 -> Füllstand B106/1
  Demux29/3 -> V911_Zulauf_zu_ZWL_geschlossen/1, Füllstand B121/1
  Bitwise AND14/1 -> Compare To Constant14/1
  Byte Reversal105/1 -> pH_QI502/1, QI502_pH_Messung_in_B504/1
  Demux16/1 -> pH_Drucksensor_Druckluft/1, Füllstand B80/1
  Demux9/6 -> Füllstand B28/1
  Byte Unpack/8 -> Demux15/1
  Demux18/5 -> Byte Reversal106/1
  Byte Unpack/11 -> Demux22/1
  Demux16/7 -> Fuellstand_Min_B503/1, Füllstand B71/1
  Demux3/2 -> MTL_Notaus/1, Füllstand B1/1
  Demux20/1 -> ZWL_Drucksensor_druckluft/1, Füllstand B96/1
  Demux7/1 -> Byte Reversal89/1
  Demux24/7 -> V702_Ruecklauf_geoeffnet/1, Füllstand B103/1
  Demux19/1 -> Byte Reversal108/1
  Demux28/7 -> V911_Zulauf_zu_REH_geschlossen/1, Füllstand B119/1
  Compare To Constant1/1 -> Demux2/1
  Demux8/8 -> V205_Stellung_intern/1, Füllstand B24/1
  Demux23/1 -> Byte Reversal113/1
  Demux6/1 -> Byte Reversal81/1
  Demux30/7 -> Füllstand B39/1
  Byte Reversal111/1 -> Durchfluss_FI1/1, WI620_Gewichtsmessung/1
  Demux20/7 -> V605_Stellung_intern/1, Füllstand B87/1
  Byte Unpack/4 -> Demux7/1
  Compare To Constant8/1 -> Demux16/1
  Compare To Constant2/1 -> Demux3/1
  Demux20/6 -> Durchflussmessung_Grenzwert_FIC601/1, Füllstand B86/1
  Demux25/3 -> Füllstand B105/1
  Byte Reversal107/1 -> Bitwise AND9/1
  Demux14/1 -> Byte Reversal96/1
  Byte Reversal101/1 -> Bitwise AND6/1
  Demux20/2 -> Fuellstand_Max_B601/1, Füllstand B82/1
  Demux18/3 -> Byte Reversal105/1
  Bitwise AND6/1 -> Compare To Constant6/1
  Byte Reversal116/1 -> Durchfluss_FI701/1, FI701_Durchflussmessung/1
  Byte Reversal100/1 -> Bitwise AND7/1
  Demux18/2 -> Byte Reversal104/1
  Demux16/3 -> V504_Stellung_Nachfolger/1, Füllstand B67/1
  Demux31/1 -> Byte Reversal121/1
  Bitwise AND1/1 -> Compare To Constant1/1
  Bitwise AND7/1 -> Compare To Constant7/1
  Demux29/1 -> V911_Zulauf_zu_pH_geschlossen/1, Füllstand B127/1
  Demux1/5 -> Fuellstand_Min_B301/1, Füllstand B44/1
  Demux2/3 -> Fuellstand_Min_B101/1, Füllstand B11/1
  Demux28/5 -> V911_Zulauf_zu_KMP_geschlossen/1, Füllstand B117/1
  Demux19/2 -> Byte Reversal107/1
  Demux18/4 -> Byte Reversal103/1
  Byte Reversal106/1 -> pH_AI_QI502/1, AI_pH_QI502_PB_DATABASE/1
  Demux29/7 -> Füllstand B125/1
  Byte Reversal114/1 -> Fuellstand_B701/1, B701_Fuellstand_B701_LI701/1
  Demux15/1 -> Byte Reversal101/1
  Demux28/6 -> V911_Zulauf_zu_KMP_geöffnet/1, Füllstand B118/1
  Demux13/4 -> V411_Stellung_VBS/1, Füllstand B58/1
  Byte Unpack/14 -> Demux27/1
  Demux29/4 -> V911_Zulauf_zu_ZWL_geoeffnet/1, Füllstand B122/1
  UDP Receive1/1 -> Byte Unpack/1
  Compare To Constant12/1 -> Demux24/1
  Demux25/2 -> Füllstand B97/1
  Demux2/7 -> Füllstand B15/1, Durchfluss_FIC101_Grenzwert/1
  Demux13/8 -> Füllstand B62/1
  Demux22/1 -> Byte Reversal109/1
  Demux4/1 -> Byte Reversal80/1
  Demux25/5 -> Füllstand B107/1
  Demux6/4 -> Byte Reversal82/1
  Demux21/3 -> Füllstand B89/1
  Demux16/5 -> Fuellstand_Min_B501/1, Füllstand B69/1
  Bitwise AND15/1 -> Compare To Constant15/1
  Byte Unpack/5 -> Demux10/1
  Demux17/7 -> Füllstand B77/1
  Demux8/6 -> Füllstand B22/1, KMP_Drucksensor_Gas_Schwellwert/1
  Demux28/3 -> V911_Zulauf_zu_MTL_geschlossen/1, Füllstand B115/1
  Demux6/2 -> Byte Reversal86/1
  Byte Reversal110/1 -> Durchfluss_FI601/1, FI601_Durchflussmessung/1
  Demux24/1 -> RCY_Drucksensor_Druckluft/1, Füllstand B112/1
  Demux9/1 -> V205_Stellung_VBS/1, Füllstand B31/1
  Demux2/4 -> V102_Ablauf_zu_KMP_VBS_geschlossen/1, Füllstand B12/1
  Byte Unpack/9 -> Demux18/1
  Demux21/6 -> Füllstand B92/1
  Demux30/4 -> Füllstand B36/1
  Demux13/7 -> Füllstand B61/1
  Demux12/3 -> Nieder_Hochdruck_Schalter_Niederdruck/1, Füllstand B51/1
  Demux5/1 -> Byte Reversal123/1
  Byte Reversal97/1 -> Temperatur_TI401/1, Temperature TI401/1
  Bitwise AND9/1 -> Compare To Constant9/1
  Demux1/7 -> V305_Stellung_Folgestation_in/1, Füllstand B46/1
  Byte Unpack/13 -> Demux26/1
  Demux17/1 -> Durchfluss_Grenzwert_FIC501/1, Füllstand B79/1
  Byte Reversal84/1 -> Fuellstand_B101/1, B101_Fuellstand/1
  Demux24/3 -> V701_Zulauf_B701_geoeffnet/1, Füllstand B99/1
  Byte Reversal124/1 -> Data Type Conversion/1, year/1  "year"
  Byte Unpack/17 -> Byte Reversal124/1
  Byte Reversal130/1 -> Data Type Conversion6/1, T501_Temperatur8/1  "second"
  Byte Reversal127/1 -> Data Type Conversion3/1, T501_Temperatur5/1  "weekday"
  Demux/3 -> Byte Reversal127/1
  Demux/5 -> Byte Reversal129/1
  Byte Reversal128/1 -> Data Type Conversion4/1, T501_Temperatur6/1  "hour"
  Demux/6 -> Byte Reversal130/1
  Demux/4 -> Byte Reversal128/1
  Demux/2 -> Byte Reversal126/1
  Demux/1 -> Byte Reversal125/1
  Byte Reversal125/1 -> Data Type Conversion1/1, T501_Temperatur3/1  "month"
  Byte Reversal126/1 -> Data Type Conversion2/1, T501_Temperatur4/1  "day"
  Byte Reversal129/1 -> Data Type Conversion5/1, T501_Temperatur7/1  "minute"
  Byte Reversal131/1 -> Demux/1
  Byte Unpack/18 -> Byte Reversal131/1
  Byte Unpack/19 -> Byte Reversal132/1
  Byte Reversal132/1 -> Data Type Conversion7/1, nanosecond/1  "nanosecond"
  Byte Reversal102/1 -> Fuellstand_B501/1, B501_Fuellstand/1
  Demux28/2 -> VBS_Notaus/1, Füllstand B114/1
  Byte Reversal199/1 -> Mux30/8
  Byte Reversal139/1 -> Mux28/8
  Byte Reversal162/1 -> Mux24/4
  Mux15/1 -> Byte Pack1/8
  Byte Reversal202/1 -> Mux2/3
  V921_Zulauf_KMP/1 -> Byte Reversal209/1
  V602_Ablauf_Kuehlbehaeler_oeffnen/1 -> Byte Reversal186/1
  Nicht belegt 23/1 -> Byte Reversal196/1
  Byte Reversal161/1 -> Mux24/3
  Mux33/1 -> Byte Pack1/5
  W303_aktivieren/1 -> Byte Reversal160/1
  Product9/1 -> Vektor Summe9/1
  V206_Wasser_Stellwert/1 -> Byte Reversal210/1
  V107_zu_KMP_VBS/1 -> Byte Reversal188/1
  Byte Reversal179/1 -> Mux26/1
  Mux29/1 -> Byte Pack1/1
  R304_Stellwert/1 -> Byte Reversal158/1
  Product11/1 -> Vektor Summe11/1
  Byte Reversal171/1 -> Mux25/3
  Byte Vektor9/1 -> Product9/2
  Byte Vektor12/1 -> Product12/2
  Vektor Summe8/1 -> Mux12/1
  Byte Reversal205/1 -> Mux2/6
  Byte Reversal168/1 -> Byte Pack1/7
  ? -> Mux3/2
  Byte Pack1/1 -> UDP Send2/1
  Vektor Summe9/1 -> Mux3/1
  Byte Reversal177/1 -> Mux30/6
  Byte Reversal200/1 -> Mux1/7
  R504_Stellwert/1 -> Byte Reversal178/1
  Byte Reversal183/1 -> Mux27/4
  Mux27/1 -> Product13/1
  Mux14/1 -> Byte Pack1/6
  Byte Reversal198/1 -> Mux1/6
  V106_offen/1 -> Byte Reversal134/1
  Mux30/1 -> Product9/1
  Byte Reversal207/1 -> Mux2/8
  Vektor Summe14/1 -> Mux18/1
  Fuellbit/1 -> Byte Reversal138/1
  V101_offen/1 -> Byte Reversal211/1
  ? -> Mux18/2
  Byte Reversal155/1 -> Mux30/5
  V503_Lauge/1 -> Byte Reversal173/1
  Byte Reversal166/1 -> Mux29/1
  V306_Stellung_extern/1 -> Byte Reversal153/1
  Byte Reversal181/1 -> Mux25/2
  Product10/1 -> Vektor Summe10/1
  Mux24/1 -> Product11/1
  V931_Zulauf_REH/1 -> Byte Reversal204/1
  Mux25/1 -> Product12/1
  Mux26/1 -> Byte Pack1/9
  Byte Reversal165/1 -> Mux24/7
  Byte Reversal211/1 -> Mux28/2
  Mux2/1 -> Product15/1
  Byte Reversal140/1 -> Mux31/3
  Byte Reversal189/1 -> Mux27/6
  Byte Reversal142/1 -> Mux29/2
  Byte Reversal148/1 -> Mux30/1
  R304_aktivieren/1 -> Byte Reversal151/1
  Byte Reversal174/1 -> Mux25/6
  V207_Ruecklauf_zu_B201/1 -> Byte Reversal149/1
  V204_nach_Druckbehaelter_drehen/1 -> Byte Reversal177/1
  ? -> Mux15/2
  Mux3/1 -> Byte Pack1/4
  V406_kuehlen_klein/1 -> Byte Reversal162/1
  Byte Reversal143/1 -> Mux29/3
  Byte Reversal172/1 -> Mux25/4
  V211_Gas_aktivieren/1 -> Byte Reversal155/1
  P301_Stellwert/1 -> Byte Reversal157/1
  Byte Reversal184/1 -> Mux27/5
  Byte Reversal185/1 -> Byte Pack1/11
  Byte Reversal188/1 -> Mux28/1
  Kuehlkreislauf_aktiv/1 -> Byte Reversal170/1
  Byte Reversal160/1 -> Mux32/2
  Byte Reversal153/1 -> Mux32/6
  Fuellbit1/1 -> Byte Reversal139/1
  Mux28/1 -> Product8/1
  Product15/1 -> Vektor Summe15/1
  Byte Reversal141/1 -> Mux31/1
  P501_Stellwert/1 -> Byte Reversal179/1
  Byte Reversal151/1 -> Mux32/4
  ? -> Mux12/2
  ? -> Mux16/2
  Byte Reversal159/1 -> Mux32/1
  Mux12/1 -> Byte Pack1/2
  V505_Stellung_VBS1/1 -> Byte Reversal175/1
  Mux18/1 -> Byte Pack1/14
  Byte Reversal210/1 -> Mux31/2
  Byte Vektor15/1 -> Product15/2
  Mux17/1 -> Byte Pack1/12
  Nicht belegt 20/1 -> Byte Reversal189/1
  pH_Regler_schalten_hold/1 -> Byte Reversal180/1
  Byte Reversal167/1 -> Mux24/8
  V911_Zulauf_MTL/1 -> Byte Reversal208/1
  P701_Stellwert/1 -> Byte Reversal193/1
  Product14/1 -> Vektor Summe14/1
  V406_kuehlen_gross/1 -> Byte Reversal164/1
  Vektor Summe13/1 -> Mux17/1
  Mux16/1 -> Byte Pack1/10
  Byte Reversal209/1 -> Mux2/2
  Byte Reversal193/1 -> Byte Pack1/13
  V205_nach_VBS_drehen/1 -> Byte Reversal147/1
  ? -> Mux19/2
  Vektor Summe12/1 -> Mux16/1
  Byte Reversal194/1 -> Mux1/1
  Byte Reversal158/1 -> Mux33/2
  Byte Reversal206/1 -> Mux2/7
  Product12/1 -> Vektor Summe12/1
  P602_Abfuellen_aktiv/1 -> Byte Reversal183/1
  Byte Reversal163/1 -> Mux24/5
  V951_Zulauf_PH/1 -> Byte Reversal205/1
  V406_kuehlen_mittel/1 -> Byte Reversal163/1
  Vektor Summe15/1 -> Mux19/1
  V305_Stellung_VBS/1 -> Byte Reversal156/1
  Byte Reversal157/1 -> Mux33/1
  R504_aktivieren/1 -> Byte Reversal171/1
  Nicht belegt 14/1 -> Byte Reversal198/1
  ? -> Mux14/2
  ? -> Mux17/2
  Mux1/1 -> Product14/1
  V961_Zulauf_ZWL/1 -> Byte Reversal206/1
  Mux32/1 -> Product10/1
  Byte Reversal138/1 -> Mux28/7
  Byte Reversal176/1 -> Mux25/8
  V971_Zulauf_RCY/1 -> Byte Reversal207/1
  V206_Wasser_aktivieren/1 -> Byte Reversal144/1
  P301_aktivieren/1 -> Byte Reversal150/1
  Byte Reversal178/1 -> Mux26/2
  Nicht belegt 21/1 -> Byte Reversal190/1
  Byte Reversal137/1 -> Mux28/6
  V504_Stellung_Nachfolgestation/1 -> Byte Reversal174/1
  P401_aktiv/1 -> Byte Reversal161/1
  Byte Reversal173/1 -> Mux25/5
  P501_aktiv/1 -> Byte Reversal181/1
  P201_Stellwert/1 -> Byte Reversal141/1
  Byte Reversal197/1 -> Mux1/5
  V202_Ablauf_zu_REH/1 -> Byte Reversal148/1
  V307_Zulauf_REK_oeffnen/1 -> Byte Reversal152/1
  Byte Reversal164/1 -> Mux24/6
  Byte Vektor14/1 -> Product14/2
  P601_aktiv/1 -> Byte Reversal182/1
  Byte Reversal144/1 -> Mux30/4
  V305_zu_umwaelzen_oeffnen/1 -> Byte Reversal159/1
  Byte Reversal204/1 -> Mux2/5
  Byte Reversal169/1 -> Mux24/1
  Vektor Summe10/1 -> Mux14/1
  Mux19/1 -> Byte Pack1/15
  P601_Stellwert/1 -> Byte Reversal185/1
  Nicht belegt 19/1 -> Byte Reversal176/1
  Byte Reversal145/1 -> Mux29/4
  Nicht belegt 16/1 -> Byte Reversal201/1
  P901_Aktivierung/1 -> Byte Reversal203/1
  Byte Reversal190/1 -> Mux27/7
  Byte Reversal149/1 -> Mux30/2
  Byte Reversal136/1 -> Mux28/5
  V605_Stellung_VBS1/1 -> Byte Reversal184/1
  P201_aktivieren/1 -> Byte Reversal133/1
  V702_Ruecklauf_zu_B701/1 -> Byte Reversal192/1
  Nicht belegt 24/1 -> Byte Reversal197/1
  Byte Reversal196/1 -> Mux1/4
  Byte Reversal191/1 -> Mux27/8
  Byte Reversal152/1 -> Mux32/5
  V402_Ablauf_Kuehlbehaelter_oeffnen/1 -> Byte Reversal169/1
  Byte Vektor10/1 -> Product10/2
  Byte Reversal180/1 -> Mux25/1
  Byte Reversal146/1 -> Mux29/5
  V411_VBS_drehen/1 -> Byte Reversal167/1
  Byte Reversal133/1 -> Mux30/3
  Byte Reversal195/1 -> Mux1/2
  Byte Reversal192/1 -> Mux1/3
  V604_Ruecklauf/1 -> Byte Reversal187/1
  Byte Reversal208/1 -> Mux2/1
  Product13/1 -> Vektor Summe13/1
  Byte Reversal201/1 -> Mux1/8
  Nicht belegt 18/1 -> Byte Reversal199/1
  Byte Reversal187/1 -> Mux27/2
  Byte Reversal135/1 -> Mux28/4
  P401_Stellwert/1 -> Byte Reversal168/1
  Byte Reversal154/1 -> Mux32/7
  V304_Stellung_extern/1 -> Byte Reversal154/1
  V502_Saeure/1 -> Byte Reversal172/1
  P102_Aktivierung/1 -> Byte Reversal137/1
  Mux31/1 -> Byte Pack1/3
  Byte Vektor11/1 -> Product11/2
  Byte Vektor13/1 -> Product13/2
  P701_aktiv/1 -> Byte Reversal194/1
  Byte Reversal147/1 -> Mux30/7
  Byte Reversal175/1 -> Mux25/7
  V941_Zulauf_REK/1 -> Byte Reversal202/1
  V211_Gas_Stellwert/1 -> Byte Reversal140/1
  Vektor Summe11/1 -> Mux15/1
  Nicht belegt 15/1 -> Byte Reversal200/1
  Product8/1 -> Vektor Summe8/1
  Byte Reversal150/1 -> Mux32/3
  V405_VBS_drehen/1 -> Byte Reversal165/1
  Byte Reversal186/1 -> Mux27/1
  V701_Zulauf_B701/1 -> Byte Reversal195/1
  Byte Vektor8/1 -> Product8/2
  Byte Reversal182/1 -> Mux27/3
  Nicht belegt 22/1 -> Byte Reversal191/1
  V105_zu_VBS/1 -> Byte Reversal136/1
  Byte Reversal134/1 -> Mux28/3
  Byte Reversal203/1 -> Mux2/4
  Byte Reversal156/1 -> Mux32/8
  Byte Reversal170/1 -> Mux24/2
  P101_Stellwert/1 -> Byte Reversal166/1
  V101_Stellwert/1 -> Byte Reversal142/1
  V106_Aktivierung/1 -> Byte Reversal145/1
  V106_Stellwert/1 -> Byte Reversal143/1
  P101_Aktivierung/1 -> Byte Reversal135/1
  P102_Stellwert/1 -> Byte Reversal146/1

== matlab function PI_v3/MATLAB Function ==
  data: ref input; ITAE output; meas input; time input
function ITAE  = fcn(ref, meas,time)
    ITAE = abs(ref-meas)*time;
end

== matlab function PI_v3/ShedulingStateMachine1 ==
  data: stopExperiment output; time input; notAusActive input; earlyStoppingActivated input; enableControl output; sollVals output size=[3]; stateOut output; V101_ref parameter; Parameters parameter
function [stopExperiment, enableControl, sollVals, stateOut] = fcn( time, notAusActive,earlyStoppingActivated, V101_ref, Parameters)
persistent state
persistent lastTransTime
% possible states:
% 1: wait for emptying of tanks
% 2: set new context and adjust valves
% 3: experiment running
% 4: stopping
% 5: stopped
if isempty(state) || time < 0.1
    state = 1;
    lastTransTime = time;
end
newState = state;

stopExperiment = false;
enableControl = false;
sollVals = [0 0 100]';

% handle transitions

if state == 1
    if time - lastTransTime  >= Parameters.idleTime
        newState = 2;
        lastTransTime = time;
    end
elseif state == 2
    if time - lastTransTime  >= Parameters.changeValTime
        newState = 3;
        lastTransTime = time;
    end
elseif state == 3
    if notAusActive || time - lastTransTime  >= Parameters.expTime || earlyStoppingActivated
        newState = 4;
        lastTransTime = time;
    end
elseif state == 4
    if time - lastTransTime  >= Parameters.stoppingTime 
        newState = 5;
        lastTransTime = time;
    end
end


state = newState;



if state == 1
    enableControl = false;
    sollVals = [0 0 100]';
    stopExperiment = false;
elseif state == 2
    enableControl = false;
    sollVals = [0 V101_ref 44.7]';
    stopExperiment = false;
elseif state == 3
    enableControl = true;
    sollVals = [0 V101_ref 44.7]';
    stopExperiment = false;
elseif state == 4
    enableControl = false;
    sollVals = [0 0 100]';
    stopExperiment = false;
elseif state == 5
    enableControl = false;
    sollVals = [0 0 100]';
    stopExperiment = true;
end



stateOut = state;
end
